simulink model "sads_balance_cubemodel"  (R2024b)
settings: Solver=FixedStepAuto  StartTime=0.0  StopTime=inf  FixedStep=0.10  RelTol=1e-3  EnableMultiTasking=on
model workspace (MAT data in the model file):
  STEPS_PER_REV = 3200
  TRAVEL_LIMIT = 22400
  starting_x = 0
  starting_y = 4800
undefined symbols (not defined in the file or in its folder): bits, DiscIntNeverNeededParam
libraries: stm32blockslib x6, simulink_extras x1, sharedtransform x1, matrix_library x1, aerolibutil x1
settings Model: STM32="{\"HardwareInterrupt\":{\"ID\":\"stm32_hwi_gettingstarted:47\"},\"DigitalPortWrite\":{\"ID\":\"stm32_hwi_gettingstarted:48\"},\"I2CControllerRead\":[{\"ID\":\"sads_balance_cubemodel:191\"},{\"ID\":\"sads_balance_cubemodel:194\"},{\"ID\":\"sads_balance_cubemodel:395\"}],\"I2CControllerWrite\":[{\"ID\":\"sads_balance_cubemodel:275\"},{\"ID\":\"sads_balance_cubemodel:332\"}],\"UARTWrite\":{\"ID\":\"sads_balance_cubemodel:374\"}}"  ParameterArgumentNames=STEPS_PER_REV  Creator=The MathWorks, Inc.  LastModifiedBy=camer
settings SolverCC: AutoInsertRateTranBlk=on
settings OptimizationCC: EnhancedBackFolding=on  PassReuseOutputArgsAs=Individual arguments  ZeroExternalMemoryAtStartup=off  ZeroInternalMemoryAtStartup=off  MaxStackSize=512  OptimizeBlockOrder=speed  DifferentSizesBufferReuse=on  OptimizationCustomize=off  EfficientTunableParamExpr=on
settings DebuggingCC: ParameterTunabilityLossMsg=error  UnconnectedInputMsg=warning  UnconnectedOutputMsg=warning  UnconnectedLineMsg=warning  SubsystemReferenceDiagnosticForUnitTest=warning
settings HardwareCC: ProdBitPerPointer=32  ProdBitPerSizeT=32  ProdBitPerPtrDiffT=32  ProdLargestAtomicInteger=Long  ProdLargestAtomicFloat=Double  ProdWordSize=32  ProdLongLongMode=on  ProdHWDeviceType=ARM Compatible->ARM Cortex
settings ModelReferenceCC: EnableRefExpFcnMdlSchedulingChecks=on
settings SFSimCC: MATLABDynamicMemAlloc=off
settings RTWCC: Description=Embedded Coder  SystemTargetFile=ert.tlc  HardwareBoard=STM32F4xx Based  TemplateMakefile=ert_default_tmf  Toolchain=GNU Tools for ARM Embedded Processors  GPUComputeCapability=3.5  DLArmComputeVersion=19.05
settings CodeAppCC: ForceParamTrailComments=on  IgnoreCustomStorageClasses=off  OperatorAnnotations=on  SimulinkDataObjDesc=on  SFDataObjDesc=on  InsertBlockDesc=on
settings ERTTargetCC: CodeReplacementLibrary=ARM Cortex-M  ExtModeTransport=3  ExtModeStaticAlloc=on  ExtModeStaticAllocSize=8000  ExtModeMexFile=ext_xcp  ExtModeIntrfLevel=Level2 - Open  InlinedParameterPlacement=Hierarchical  DynamicArrayContainerType=coder::array

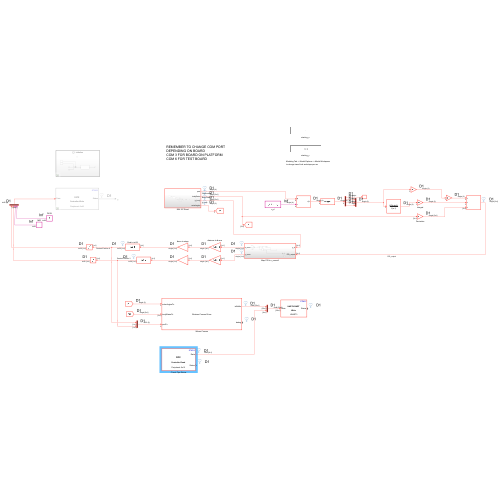
[thumbnail: Simulink's stored preview of the top-level diagram]
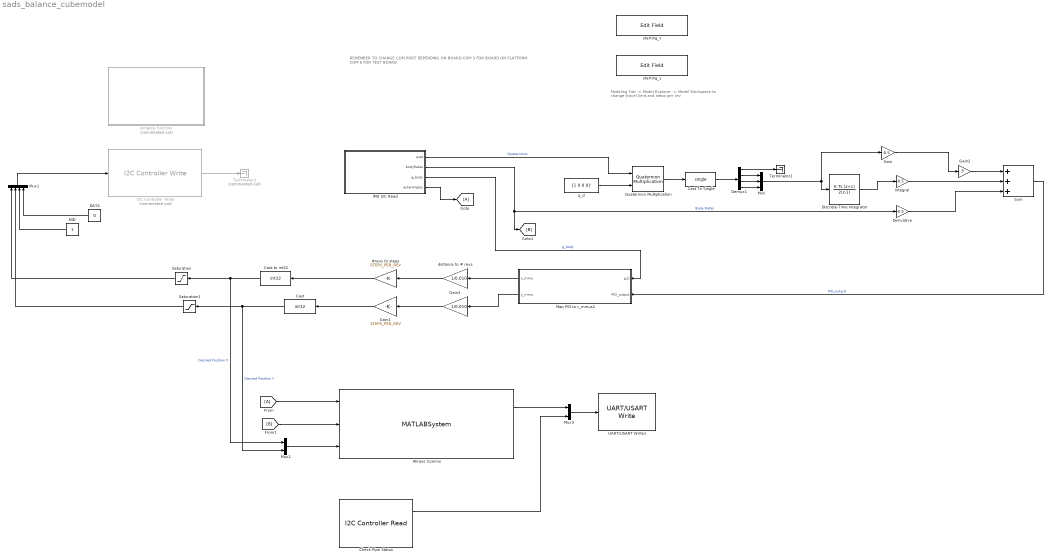
== system sads_balance_cubemodel ==
  note: Modeling Tab -> Model Explorer -> Model Workspace
      | to change travel limit and steps per rev
  note: REMEMBER TO CHANGE COM PORT DEPENDING ON BOARD
      | COM 3 FOR BOARD ON PLATFORM
      | COM 6 FOR TEST BOARD
  #revs to steps : Gain  Gain=STEPS_PER_REV
  Cast : DataTypeConversion  OutDataTypeStr=int32  SaturateOnIntegerOverflow=off  RndMeth=Floor
  Cast To Single : DataTypeConversion  OutDataTypeStr=single  SaturateOnIntegerOverflow=off  RndMeth=Floor
  Cast to int32 : DataTypeConversion  OutDataTypeStr=int32  SaturateOnIntegerOverflow=off  RndMeth=Floor
  Check Pipe Status : stm32blockslib/I2C Controller Read  I2CModule=I2C2  Mode=Controller  AddressingMode=7-bits  PeripheralByteOrder=BigEndian  OwnPeripheralAddress=uint8(170)  PeripheralAddressVia=Dialog  PeripheralAddress=0x12  RegisterAddressMode=off  RegisterAddressVia=Dialog  RegisterAddress=0x12  RepeatedStart=off  NoAck=on  OutputStatus=on  BlockMode=Receive  DataType=uint8  DataLength=6  Timeout=0.100  SampleTime=-1
      settings: LibrarySourceBlock=stm32f4xxblockslib/I2C Controller Read
  DATA : Constant  Value=0  OutDataTypeStr=int32
  Demux1 : Demux
  Derivative : Gain  Gain=-0.5
  Discrete-Time Integrator : DiscreteIntegrator  IntegratorMethod=Integration: Trapezoidal  InitialCondition=[0,0,0]'  SampleTime=-1  OutDataTypeStr=single  ICPrevOutput=DiscIntNeverNeededParam  ICPrevScaledInput=DiscIntNeverNeededParam
  From : From
  Gain : Gain  Gain=-0.5  ParamDataTypeStr=single
  Gain1 : Gain  Gain=STEPS_PER_REV
  Gain2 : Gain  Gain=5
  Gain3 : Gain  Gain=1/0.010
  Goto : Goto
  I2C Controller Write : stm32blockslib/I2C Controller Write  Commented=on  I2CModule=I2C2  Mode=Controller  AddressingMode=7-bits  PeripheralByteOrder=LittleEndian  OwnPeripheralAddress=uint8(170)  PeripheralAddressVia=Dialog  PeripheralAddress=hex2dec('0x42')  RegisterAddressMode=on  RegisterAddressVia=Dialog  RegisterAddress=hex2dec('0x00')  RepeatedStart=off  NoAck=off  OutputStatus=on  BlockMode=Transmit  DataType=uint8  DataLength=1  Timeout=0.002  SampleTime=-1
      settings: LibrarySourceBlock=stm32f4xxblockslib/I2C Controller Write
  IMU I2C Read : Subsystem
  Initialize Function : Subsystem  Commented=on  TreatAsAtomicUnit=on
  Integral : Gain  Gain=-0.5
  MID : Constant  OutDataTypeStr=int32
  Map PID to r_mmus2 : Subsystem
  Mux : Mux  Inputs=3
  Mux1 : Mux
  Mux2 : Mux  Inputs=2
  Mux3 : Mux  Inputs=2
  Quaternion Multiplication : aerolibutil/Quaternion Multiplication
  Saturation : Saturate  UpperLimit=TRAVEL_LIMIT - starting_x  LowerLimit=-TRAVEL_LIMIT - starting_x
  Saturation1 : Saturate  UpperLimit=TRAVEL_LIMIT - starting_y  LowerLimit=-TRAVEL_LIMIT - starting_y
  Sum : Sum  Inputs=+++
  Terminator1 : Terminator
  Terminator2 : Terminator  Commented=on
  UART/USART Write1 : stm32blockslib/UART//USART Write  UARTModule=USART3  LengthOfDataToSend=off  BlockingMode=off  BlockingTimeout=0.1  OutputStatus=on
      settings: LibrarySourceBlock=stm32f4xxblockslib/UART//USART Write
  Wiress Comms : MATLABSystem  System=Comm_Driver_Sys_Obj
      mask Type: Comm_Driver_Sys_Obj
      mask Display:
      | disp('Wireless Comms Driver');
      | port_label('input',1,'eulerAnglesTx');
      | port_label('input',2,'bodyRatesTx');
      | port_label('input',3,'posTx');
      | port_label('output',1,'txBuffer');
      | port_label('output',2,'debug');
  distance to # revs : Gain  Gain=1/0.010
  q_d : Constant  Value=[1 0 0 0]'  OutDataTypeStr=single
  starting_x : EditField  LabelPosition=Hide  ShowInitialText=on  Alignment=Center
  starting_y : EditField  LabelPosition=Hide  ShowInitialText=on  Alignment=Center
  wires:
  Cast to int32/1 -> Mux2/1, Saturation/1  "Desired Position X"
  IMU I2C Read/3(g_body) -> Map PID to r_mmus2/1(g_b)  "g_body"
  IMU I2C Read/1(quat) -> Quaternion Multiplication/1  "Quaternions"
  IMU I2C Read/2(bodyRates) -> Derivative/1, [B]  "Body Rates"
  q_d/1 -> Quaternion Multiplication/2
  Quaternion Multiplication/1 -> Cast To Single/1
  Demux1/2 -> Mux/1
  Demux1/3 -> Mux/2
  Demux1/4 -> Mux/3
  Mux/1 -> Gain/1, Discrete-Time Integrator/1
  Sum/1 -> Map PID to r_mmus2/2(PID_output)  "PID_output"
  Integral/1 -> Sum/2
  Demux1/1 -> Terminator1/1
  Derivative/1 -> Sum/3
  Cast To Single/1 -> Demux1/1
  Discrete-Time Integrator/1 -> Integral/1
  Map PID to r_mmus2/1(x_mmu) -> distance to # revs/1
  Map PID to r_mmus2/2(y_mmu) -> Gain3/1
  #revs to steps/1 -> Cast to int32/1
  Gain1/1 -> Cast/1
  Cast/1 -> Mux2/2, Saturation1/1  "Desired Position Y"
  MID/1 -> Mux1/3
  DATA/1 -> Mux1/4
  Mux1/1 -> I2C Controller Write/1
  I2C Controller Write/1 -> Terminator2/1
  distance to # revs/1 -> #revs to steps/1
  Gain3/1 -> Gain1/1
  Saturation1/1 -> Mux1/2
  Saturation/1 -> Mux1/1
  Gain/1 -> Gain2/1
  Gain2/1 -> Sum/1
  Wiress Comms/1 -> Mux3/1
  From/1 -> Wiress Comms/1
  IMU I2C Read/4(eulerAngles) -> Goto/1
  [B] -> Wiress Comms/2
  Mux2/1 -> Wiress Comms/3
  Check Pipe Status/1 -> Mux3/2
  Mux3/1 -> UART/USART Write1/1

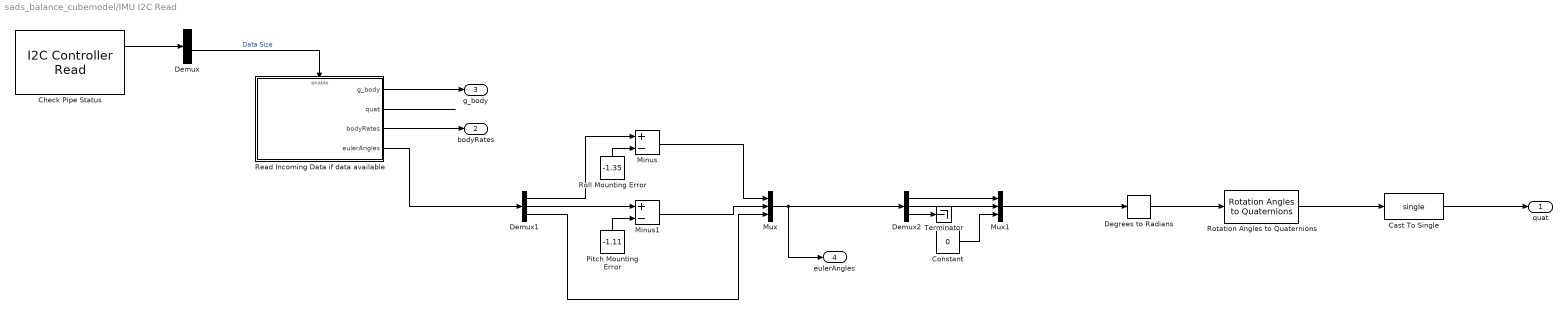
== system sads_balance_cubemodel/IMU I2C Read ==
  Cast To Single : DataTypeConversion  OutDataTypeStr=single  SaturateOnIntegerOverflow=off  RndMeth=Floor
  Check Pipe Status : stm32blockslib/I2C Controller Read  I2CModule=I2C1  Mode=Controller  AddressingMode=7-bits  PeripheralByteOrder=BigEndian  OwnPeripheralAddress=uint8(170)  PeripheralAddressVia=Dialog  PeripheralAddress=0x6B  RegisterAddressMode=on  RegisterAddressVia=Dialog  RegisterAddress=0x04  RepeatedStart=off  NoAck=off  OutputStatus=on  BlockMode=Receive  DataType=uint8  DataLength=4  Timeout=0.001  SampleTime=-1
      settings: LibrarySourceBlock=stm32f4xxblockslib/I2C Controller Read
  Constant : Constant  Value=0  OutDataTypeStr=single
  Degrees to Radians : simulink_extras/Transformations/Degrees to Radians
  Demux : Demux
  Demux1 : Demux  Outputs=3
  Demux2 : Demux  Outputs=3
  Minus : Sum  Inputs=+-
  Minus1 : Sum  Inputs=+-
  Mux : Mux  Inputs=3
  Mux1 : Mux  Inputs=3
  Pitch Mounting Error : Constant  Value=-1.11  OutDataTypeStr=single
  Read Incoming Data if data available : Subsystem  TreatAsAtomicUnit=on
  Roll Mounting Error : Constant  Value=-1.35  OutDataTypeStr=single
  Rotation Angles to Quaternions : sharedtransform/Rotation Angles to Quaternions  rotationOrder=XYZ  aMode=aMode
  Terminator : Terminator
  quat : Outport
  bodyRates : Outport  Port=2
  g_body : Outport  Port=3
  eulerAngles : Outport  Port=4
  wires:
  Read Incoming Data if data available/1(g_body) -> g_body/1
  Demux/3 -> Read Incoming Data if data available/Enable  "Data Size"
  Check Pipe Status/1 -> Demux/1
  Read Incoming Data if data available/2(quat) -> ?
  Read Incoming Data if data available/3(bodyRates) -> bodyRates/1
  Degrees to Radians/1 -> Rotation Angles to Quaternions/1
  Read Incoming Data if data available/4(eulerAngles) -> Demux1/1
  Mux/1 -> Demux2/1, eulerAngles/1
  Demux1/1 -> Minus/1
  Demux1/2 -> Minus1/1
  Rotation Angles to Quaternions/1 -> Cast To Single/1
  Cast To Single/1 -> quat/1
  Minus/1 -> Mux/1
  Minus1/1 -> Mux/2
  Roll Mounting Error/1 -> Minus/2
  Pitch Mounting Error/1 -> Minus1/2
  Demux1/3 -> Mux/3
  Demux2/1 -> Mux1/1
  Demux2/2 -> Mux1/2
  Mux1/1 -> Degrees to Radians/1
  Constant/1 -> Mux1/3
  Demux2/3 -> Terminator/1

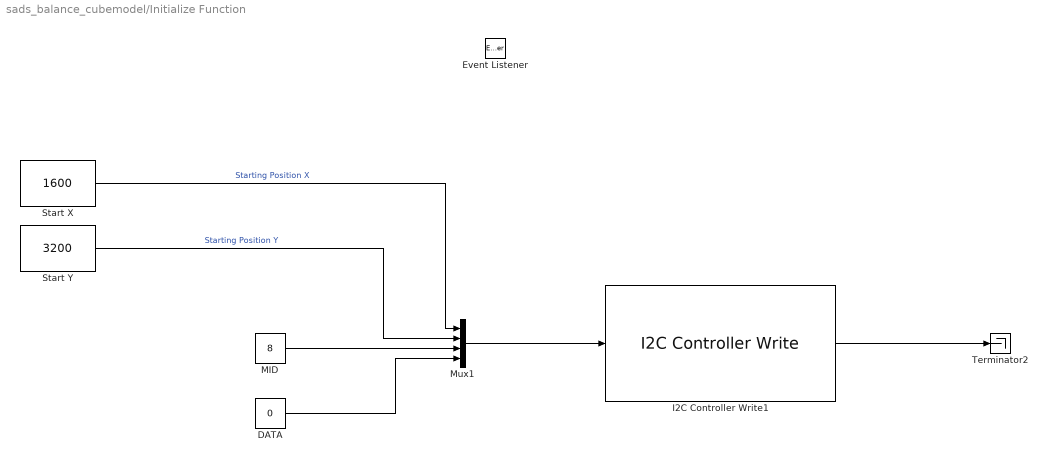
== system sads_balance_cubemodel/Initialize Function ==
  DATA : Constant  Value=0  OutDataTypeStr=int32
  Event Listener : EventListener  DisableCoverage=on  EventName=reset
  I2C Controller Write1 : stm32blockslib/I2C Controller Write  I2CModule=I2C2  Mode=Controller  AddressingMode=7-bits  PeripheralByteOrder=LittleEndian  OwnPeripheralAddress=uint8(170)  PeripheralAddressVia=Dialog  PeripheralAddress=hex2dec('0x42')  RegisterAddressMode=on  RegisterAddressVia=Dialog  RegisterAddress=hex2dec('0x00')  RepeatedStart=off  NoAck=off  OutputStatus=on  BlockMode=Transmit  DataType=uint8  DataLength=1  Timeout=0.100  SampleTime=-1
      settings: LibrarySourceBlock=stm32f4xxblockslib/I2C Controller Write
  MID : Constant  Value=8  OutDataTypeStr=int32
  Mux1 : Mux
  Start X : Constant  Value=1600  OutDataTypeStr=int32
  Start Y : Constant  Value=3200  OutDataTypeStr=int32
  Terminator2 : Terminator
  wires:
  MID/1 -> Mux1/3
  Start Y/1 -> Mux1/2  "Starting Position Y"
  Mux1/1 -> I2C Controller Write1/1
  Start X/1 -> Mux1/1  "Starting Position X"
  DATA/1 -> Mux1/4
  I2C Controller Write1/1 -> Terminator2/1

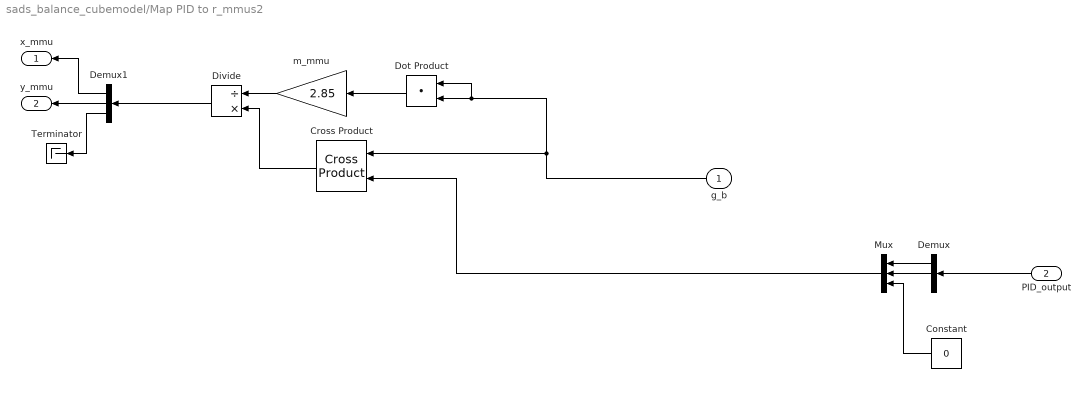
== system sads_balance_cubemodel/Map PID to r_mmus2 ==
  g_b : Inport
  PID_output : Inport  Port=2
  Constant : Constant  Value=0  OutDataTypeStr=single
  Cross Product : matrix_library/Cross Product
  Demux : Demux  Outputs=3
  Demux1 : Demux  Outputs=3
  Divide : Product  Inputs=/*
  Dot Product : DotProduct  OutDataTypeStr=Inherit: Inherit via internal rule
  Mux : Mux  Inputs=3
  Terminator : Terminator
  m_mmu : Gain  Gain=2.85
  x_mmu : Outport
  y_mmu : Outport  Port=2
  wires:
  PID_output/1 -> Demux/1
  g_b/1 -> Dot Product/1, Dot Product/2, Cross Product/1
  Demux/2 -> Mux/2
  Demux/1 -> Mux/1
  Constant/1 -> Mux/3
  Mux/1 -> Cross Product/2
  Dot Product/1 -> m_mmu/1
  m_mmu/1 -> Divide/1
  Cross Product/1 -> Divide/2
  Divide/1 -> Demux1/1
  Demux1/3 -> Terminator/1
  Demux1/1 -> x_mmu/1
  Demux1/2 -> y_mmu/1

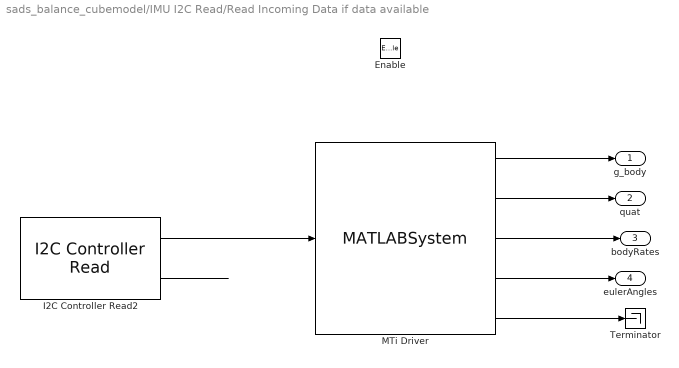
== system sads_balance_cubemodel/IMU I2C Read/Read Incoming Data if data available ==
  Enable : EnablePort
  I2C Controller Read2 : stm32blockslib/I2C Controller Read  I2CModule=I2C1  Mode=Controller  AddressingMode=7-bits  PeripheralByteOrder=BigEndian  OwnPeripheralAddress=uint8(170)  PeripheralAddressVia=Dialog  PeripheralAddress=0x6B  RegisterAddressMode=on  RegisterAddressVia=Dialog  RegisterAddress=0x06  RepeatedStart=off  NoAck=off  OutputStatus=on  BlockMode=Receive  DataType=uint8  DataLength=91  Timeout=0.001  SampleTime=-1
  MTi Driver : MATLABSystem  System=MTi_Driver_Sys_Obj
      mask Type: MTi_Driver_Sys_Obj
      mask Display:
      | disp('MTi Driver');
      | port_label('input',1,'bytesIn');
      | port_label('output',1,'g_body');
      | port_label('output',2,'quat');
      | port_label('output',3,'bodyRates');
      | port_label('output',4,'eulerAngles');
      | port_label('output',5,'debug');
  Terminator : Terminator
  g_body : Outport
  quat : Outport  Port=2
  bodyRates : Outport  Port=3
  eulerAngles : Outport  Port=4
  wires:
  I2C Controller Read2/1 -> MTi Driver/1
  MTi Driver/1 -> g_body/1
  MTi Driver/2 -> quat/1
  MTi Driver/3 -> bodyRates/1
  MTi Driver/5 -> Terminator/1
  MTi Driver/4 -> eulerAngles/1
  I2C Controller Read2/2 -> ?
